simulink model "upravljanjePozicijom2012a"  (R2012a)
settings: Solver=ode3  SolverMode=SingleTasking  StartTime=0.0  StopTime=100  RelTol=1e-3
values from neighbouring files (symbols this model uses):
  a = 0.8    [konstantePozicija.m]
  b = 0.7    [konstanteBrzina.m]    (also in konstantePozicija.m = 1)
  c = 140    [konstantePozicija.m]
  K3 = 3    [konstantePozicija.m]
  K4 = 5    [konstantePozicija.m]
  N = 3    [konstanteBrzina.m]    (also in konstantePozicija.m = 8)
  T = 0.01    [konstanteBrzina.m]    (also in konstantePozicija.m)
  Td3 = 0.3    [konstantePozicija.m]
  Td4 = 0.1    [konstantePozicija.m]
  Ti4 = 1.1    [konstantePozicija.m]
settings Model: CovMetricSettings=dwe  CovHtmlReporting=off  covSaveCumulativeToWorkspaceVar=off  CovSaveSingleToWorkspaceVar=off  CovExternalEMLEnable=on  Creator=Anja  LastModifiedBy=Anja
settings DataIOCC: SaveFormat=StructureWithTime  ReturnWorkspaceOutputs=off
settings OptimizationCC: LifeSpan=inf  SimCompilerOptimization=Off
settings DebuggingCC: FcnCallInpInsideContextMsg=Enable All
settings HardwareCC: ProdWordSize=32  ProdHWDeviceType=Specified
settings SFSimCC: SimUseLocalCustomCode=off
settings RTWCC: RTWUseLocalCustomCode=off  RTWCompilerOptimization=Off
settings GRTTargetCC: CodeReplacementLibrary=C99 (ISO)  CPPClassGenCompliant=off

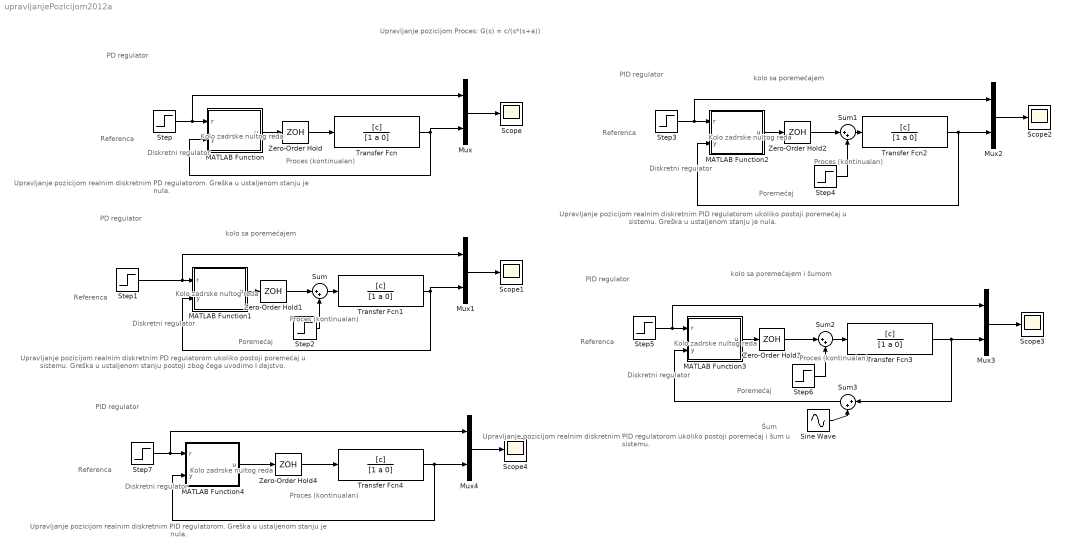
== system upravljanjePozicijom2012a ==
  note: Upravljanje pozicijom
      | Proces: G(s) = c/(s*(s+a))
  note: PD regulator
  note: PD regulator
  note: kolo sa poremećajem
  note: PID regulator
  note: kolo sa poremećajem
  note: PID regulator
  note: kolo sa poremećajem i šumom
  note: Upravljanje pozicijom realnim diskretnim PD regulatorom. Greška u ustaljenom stanju je nula.
  note: Upravljanje pozicijom realnim diskretnim PD regulatorom ukoliko postoji poremećaj u sistemu. Greška u ustaljenom stanju postoji zbog čega uvodimo I dejstvo.
  note: Upravljanje pozicijom realnim diskretnim PID regulatorom ukoliko postoji poremećaj u sistemu. Greška u ustaljenom stanju je nula.
  note: Upravljanje pozicijom realnim diskretnim PID regulatorom ukoliko postoji poremećaj i šum u sistemu.
  note: Upravljanje pozicijom realnim diskretnim PID regulatorom. Greška u ustaljenom stanju je nula.
  note: PID regulator
  note: Referenca
  note: Referenca
  note: Referenca
  note: Referenca
  note: Referenca
  note: Diskretni regulator
  note: Diskretni regulator
  note: Diskretni regulator
  note: Diskretni regulator
  note: Diskretni regulator
  note: Kolo zadrske nultog reda
  note: Kolo zadrske nultog reda
  note: Kolo zadrske nultog reda
  note: Kolo zadrske nultog reda
  note: Kolo zadrske nultog reda
  note: Proces (kontinualan)
  note: Proces (kontinualan)
  note: Proces (kontinualan)
  note: Proces (kontinualan)
  note: Proces (kontinualan)
  note: Poremećaj
  note: Poremećaj
  note: Poremećaj
  note: Šum
  MATLAB Function : MATLAB Function  TreatAsAtomicUnit=on
      settings: PermitHierarchicalResolution=ParametersOnly
  MATLAB Function1 : MATLAB Function  TreatAsAtomicUnit=on
      settings: PermitHierarchicalResolution=ParametersOnly
  MATLAB Function2 : MATLAB Function  TreatAsAtomicUnit=on
      settings: PermitHierarchicalResolution=ParametersOnly
  MATLAB Function3 : MATLAB Function  TreatAsAtomicUnit=on
      settings: PermitHierarchicalResolution=ParametersOnly
  MATLAB Function4 : MATLAB Function  TreatAsAtomicUnit=on
      settings: PermitHierarchicalResolution=ParametersOnly
  Mux{,1..4} (5 alike) : Mux  Inputs=2
  Scope{,1..4} (5 alike) : Scope
      Scope settings: TimeRange=auto  MaxDataPoints=5000  SaveToWorkspace=off  SaveName=ScopeData  YMin=1.999941  YMax=2.000009  SampleTime=-1
      Scope1 settings: TimeRange=auto  MaxDataPoints=5000  SaveToWorkspace=off  YMin=-0.255  YMax=2.295  SampleTime=-1
      Scope2 settings: TimeRange=auto  MaxDataPoints=5000  SaveToWorkspace=off  SaveName=ScopeData2  YMin=-0.25423  YMax=2.28811  SampleTime=-1
      Scope3 settings: TimeRange=auto  MaxDataPoints=5000  SaveToWorkspace=off  SaveName=ScopeData3  YMin=-1.84815  YMax=7.24007  SampleTime=-1
      Scope4 settings: TimeRange=auto  MaxDataPoints=5000  SaveToWorkspace=off  YMin=1.94244  YMax=2.01869  SampleTime=-1
  Sine Wave : Sin  Amplitude=0.05  Frequency=50000  SampleTime=0
  Step{,1,3,5,7} (5 alike) : Step  After=2  SampleTime=T
  Step2 : Step  Time=25  After=0.2  SampleTime=0
  Step4 : Step  Time=50  After=0.2  SampleTime=0
  Step6 : Step  Time=50  After=0.2  SampleTime=0
  Sum{,1..3} (4 alike) : Sum  Inputs=|++
  Transfer Fcn{,1..4} (5 alike) : TransferFcn  Numerator=[c]  Denominator=[1 a 0]
  Zero-Order Hold{,1..4} (5 alike) : ZeroOrderHold  SampleTime=T
  wires:
  MATLAB Function/1(u) -> Zero-Order Hold/1
  Step/1 -> Mux/1, MATLAB Function/1(r)
  Mux/1 -> Scope/1
  Transfer Fcn/1 -> Mux/2, MATLAB Function/2(y)
  Step1/1 -> Mux1/1, MATLAB Function1/1(r)
  Mux1/1 -> Scope1/1
  Transfer Fcn1/1 -> Mux1/2, MATLAB Function1/2(y)
  Sum/1 -> Transfer Fcn1/1
  Step2/1 -> Sum/2
  Transfer Fcn2/1 -> Mux2/2, MATLAB Function2/2(y)
  Mux2/1 -> Scope2/1
  Step3/1 -> Mux2/1, MATLAB Function2/1(r)
  Step4/1 -> Sum1/2
  MATLAB Function2/1(u) -> Zero-Order Hold2/1
  Sum1/1 -> Transfer Fcn2/1
  MATLAB Function3/1(u) -> Zero-Order Hold3/1
  Step6/1 -> Sum2/2
  Mux3/1 -> Scope3/1
  Step5/1 -> Mux3/1, MATLAB Function3/1(r)
  Transfer Fcn3/1 -> Sum3/1, Mux3/2
  Sum2/1 -> Transfer Fcn3/1
  Sine Wave/1 -> Sum3/2
  Zero-Order Hold/1 -> Transfer Fcn/1
  MATLAB Function1/1(u) -> Zero-Order Hold1/1
  Zero-Order Hold1/1 -> Sum/1
  Zero-Order Hold2/1 -> Sum1/1
  Zero-Order Hold3/1 -> Sum2/1
  Sum3/1 -> MATLAB Function3/2(y)
  Step7/1 -> Mux4/1, MATLAB Function4/1(r)
  Zero-Order Hold4/1 -> Transfer Fcn4/1
  Transfer Fcn4/1 -> Mux4/2, MATLAB Function4/2(y)
  MATLAB Function4/1(u) -> Zero-Order Hold4/1
  Mux4/1 -> Scope4/1

== matlab function upravljanjePozicijom2012a/MATLAB Function1 ==
  settings: updateMethod=DISCRETE
  data: u output; r input; y input; K3 parameter; N parameter; Td3 parameter; T parameter
function u = fcn(r, y, K3, N, Td3, T)

% implementacija realnog diskretnog PD regulatora
% Ulazni parametri su: r - referenca, y - izlaz iz sistema (procesa), K3 -
% proporcionalno pojacanje, T - perioda odabiranja, Td3 - vremenska konstanta diferenciranja, 
% N - vremenska konstanta niskopropusnog filtra, b - tezinski faktor.
% Izlazni parametar je upravljanje: u = P + D.
% D dejstvo je diskretizovano Tustinom.
%c = (2*Td2 - N*T)/(2*Td2 + N*T);
%d = 2*K2*N*Td2/(2*Td2 + N*T);
%D(kT) = c*D(kT-T) - d*(y(kT) - y(kT-T));
% Za cuvanje prethodnih vrednosti neke promenljive, izmedju poziva f-je,
% koristi se funkacije persistent. Pogledati help persistent

persistent Dp; % D(kT-T)
persistent yp; % y(kT-T)

% Inicijalizacija perzistentnih promeniljivih Dp i yp na nulu ukoliko su
% prazne (npr. na pocetku)
if (isempty(Dp))
    Dp=0;
end

if (isempty(yp))
    yp=0;
end


P = K3 * (r - y); % deo upravljanja - P dejstvo
c = (2*Td3 - N*T)/(2*Td3 + N*T); % konstanta
d = 2*K3*N*Td3/(2*Td3 + N*T); % konstanta
D = c*Dp - d*(y - yp); % D dejstvo
u = P + D; % ukupno upravljanje

%azuriranje promenljivih
Dp = D;
yp=y;

end

== matlab function upravljanjePozicijom2012a/MATLAB Function ==
  settings: updateMethod=DISCRETE
  data: u output; r input; y input; K3 parameter; N parameter; Td3 parameter; T parameter
function u = fcn(r, y, K3, N, Td3, T)

% implementacija realnog diskretnog PD regulatora
% Ulazni parametri su: r - referenca, y - izlaz iz sistema (procesa), K3 -
% proporcionalno pojacanje, T - perioda odabiranja, Td3 - vremenska konstanta diferenciranja, 
% N - vremenska konstanta niskopropusnog filtra, b - tezinski faktor.
% Izlazni parametar je upravljanje: u = P + D.
% D dejstvo je diskretizovano Tustinom.
%c = (2*Td2 - N*T)/(2*Td2 + N*T);
%d = 2*K2*N*Td2/(2*Td2 + N*T);
%D(kT) = c*D(kT-T) - d*(y(kT) - y(kT-T));
% Za cuvanje prethodnih vrednosti neke promenljive, izmedju poziva f-je,
% koristi se funkacije persistent. Pogledati help persistent

persistent Dp; % D(kT-T)
persistent yp; % y(kT-T)

% Inicijalizacija perzistentnih promeniljivih Dp i yp na nulu ukoliko su
% prazne (npr. na pocetku)
if (isempty(Dp))
    Dp=0;
end

if (isempty(yp))
    yp=0;
end


P = K3 * (r - y); % deo upravljanja - P dejstvo
c = (2*Td3 - N*T)/(2*Td3 + N*T); % konstanta
d = 2*K3*N*Td3/(2*Td3 + N*T); % konstanta
D = c*Dp - d*(y - yp); % D dejstvo
u = P + D; % ukupno upravljanje

%azuriranje promenljivih
Dp = D;
yp=y;

end

== matlab function upravljanjePozicijom2012a/MATLAB Function2 ==
  settings: updateMethod=DISCRETE
  data: u output; r input; y input; K4 parameter; N parameter; Td4 parameter; T parameter; Ti4 parameter; b parameter
function u = fcn(r, y, K4, N, Td4, T, Ti4, b)

% implementacija realnog diskretnog PID regulatora
% Ulazni parametri su: r - referenca, y - izlaz iz sistema (procesa), K4 -
% proporcionalno pojacanje, T - perioda odabiranja, Td4 - vremenska konstanta diferenciranja, 
% N - vremenska konstanta niskopropusnog filtra, b - tezinski faktor, Ti4 - vremenska
% konstantna integraljenja.
% Izlazni parametar je upravljanje: u = P + I + D.
% I dejstvo je diskretizovano diferenciranjem unazad I(kT + T) = I(kT) + (K1*T/Ti1)*e(kT)
% I(kT) = I(kT-T) + K1*T*(r(kT-T) - y(kT-T))/Ti1
% D dejstvo je diskretizovano Tustinom.
%c = (2*Td2 - N*T)/(2*Td2 + N*T);
%d = 2*K2*N*Td2/(2*Td2 + N*T);
%D(kT) = c*D(kT-T) - d*(y(kT) - y(kT-T));
% Za cuvanje prethodnih vrednosti neke promenljive, izmedju poziva f-je,
% koristi se funkacije persistent. Pogledati help persistent

persistent Ip; % I(kT-T)
persistent yp; % y(kT-T)
persistent rp; % r(kT-T)
persistent Dp; % D(kT-T)

% Inicijalizacija perzistentnih promeniljivih Ip, yp i rp na nulu ukoliko su
% prazne (npr. na pocetku)
if (isempty(Dp))
    Dp=0;
end

if (isempty(Ip))
    Ip=0;
end

if (isempty(yp))
    yp=0;
end

if (isempty(rp))
    rp=0;
end

P = K4 * (b*r - y); % P dejstvo
I = Ip + K4*T*(rp - yp)/Ti4; % I dejstvo
c = (2*Td4 - N*T)/(2*Td4 + N*T); % konstanta
d = 2*K4*N*Td4/(2*Td4 + N*T); % konstanta
D = c*Dp - d*(y - yp); % D dejstvo
u = P + I + D; % ukupno upravjanje

% azuriranje promenljivih
Dp = D;
yp=y;
rp = r;
Ip = I;

end

== matlab function upravljanjePozicijom2012a/MATLAB Function3 ==
  settings: updateMethod=DISCRETE
  data: u output; r input; y input; K4 parameter; N parameter; Td4 parameter; T parameter; Ti4 parameter; b parameter
function u = fcn(r, y, K4, N, Td4, T, Ti4, b)

% implementacija realnog diskretnog PID regulatora
% Ulazni parametri su: r - referenca, y - izlaz iz sistema (procesa), K4 -
% proporcionalno pojacanje, T - perioda odabiranja, Td4 - vremenska konstanta diferenciranja, 
% N - vremenska konstanta niskopropusnog filtra, b - tezinski faktor, Ti4 - vremenska
% konstantna integraljenja.
% Izlazni parametar je upravljanje: u = P + I + D.
% I dejstvo je diskretizovano diferenciranjem unazad I(kT + T) = I(kT) + (K1*T/Ti1)*e(kT)
% I(kT) = I(kT-T) + K1*T*(r(kT-T) - y(kT-T))/Ti1
% D dejstvo je diskretizovano Tustinom.
%c = (2*Td2 - N*T)/(2*Td2 + N*T);
%d = 2*K2*N*Td2/(2*Td2 + N*T);
%D(kT) = c*D(kT-T) - d*(y(kT) - y(kT-T));
% Za cuvanje prethodnih vrednosti neke promenljive, izmedju poziva f-je,
% koristi se funkacije persistent. Pogledati help persistent

persistent Ip; % I(kT-T)
persistent yp; % y(kT-T)
persistent rp; % r(kT-T)
persistent Dp; % D(kT-T)

% Inicijalizacija perzistentnih promeniljivih Ip, yp i rp na nulu ukoliko su
% prazne (npr. na pocetku)
if (isempty(Dp))
    Dp=0;
end

if (isempty(Ip))
    Ip=0;
end

if (isempty(yp))
    yp=0;
end

if (isempty(rp))
    rp=0;
end

P = K4 * (b*r - y); % P dejstvo
I = Ip + K4*T*(rp - yp)/Ti4; % I dejstvo
c = (2*Td4 - N*T)/(2*Td4 + N*T); % konstanta
d = 2*K4*N*Td4/(2*Td4 + N*T); % konstanta
D = c*Dp - d*(y - yp); % D dejstvo
u = P + I + D; % ukupno upravjanje

% azuriranje promenljivih
Dp = D;
yp=y;
rp = r;
Ip = I;

end

== matlab function upravljanjePozicijom2012a/MATLAB Function4 ==
  settings: updateMethod=DISCRETE
  data: u output; r input; y input; K4 parameter; N parameter; Td4 parameter; T parameter; Ti4 parameter; b parameter
function u = fcn(r, y, K4, N, Td4, T, Ti4, b)

% implementacija realnog diskretnog PID regulatora
% Ulazni parametri su: r - referenca, y - izlaz iz sistema (procesa), K4 -
% proporcionalno pojacanje, T - perioda odabiranja, Td4 - vremenska konstanta diferenciranja, 
% N - vremenska konstanta niskopropusnog filtra, b - tezinski faktor, Ti4 - vremenska
% konstantna integraljenja.
% Izlazni parametar je upravljanje: u = P + I + D.
% I dejstvo je diskretizovano diferenciranjem unazad I(kT + T) = I(kT) + (K1*T/Ti1)*e(kT)
% I(kT) = I(kT-T) + K1*T*(r(kT-T) - y(kT-T))/Ti1
% D dejstvo je diskretizovano Tustinom.
%c = (2*Td2 - N*T)/(2*Td2 + N*T);
%d = 2*K2*N*Td2/(2*Td2 + N*T);
%D(kT) = c*D(kT-T) - d*(y(kT) - y(kT-T));
% Za cuvanje prethodnih vrednosti neke promenljive, izmedju poziva f-je,
% koristi se funkacije persistent. Pogledati help persistent

persistent Ip; % I(kT-T)
persistent yp; % y(kT-T)
persistent rp; % r(kT-T)
persistent Dp; % D(kT-T)

% Inicijalizacija perzistentnih promeniljivih Ip, yp i rp na nulu ukoliko su
% prazne (npr. na pocetku)
if (isempty(Dp))
    Dp=0;
end

if (isempty(Ip))
    Ip=0;
end

if (isempty(yp))
    yp=0;
end

if (isempty(rp))
    rp=0;
end

P = K4 * (b*r - y); % P dejstvo
I = Ip + K4*T*(rp - yp)/Ti4; % I dejstvo
c = (2*Td4 - N*T)/(2*Td4 + N*T); % konstanta
d = 2*K4*N*Td4/(2*Td4 + N*T); % konstanta
D = c*Dp - d*(y - yp); % D dejstvo
u = P + I + D; % ukupno upravjanje

% azuriranje promenljivih
Dp = D;
yp=y;
rp = r;
Ip = I;

end
